simulink model "Closed_loop_response_PD_Controller"  (R2023a)
settings: Solver=FixedStepDiscrete  StartTime=0.0  StopTime=12  FixedStep=0.01  RelTol=1e-3  EnableMultiTasking=on
model workspace (MAT data in the model file):
  in = 90
undefined symbols (not defined in the file): DiscIntNeverNeededParam
libraries: M5Core_Library x2, simulink x1
settings Model: ExtModeTrigDuration=2  Creator=auw_a  LastModifiedBy=auw_a
settings OptimizationCC: EnhancedBackFolding=on  PassReuseOutputArgsAs=Individual arguments  ZeroExternalMemoryAtStartup=off  ZeroInternalMemoryAtStartup=off  MaxStackSize=64  OptimizeBlockOrder=speed  DifferentSizesBufferReuse=on  OptimizationCustomize=off  EfficientTunableParamExpr=on
settings DebuggingCC: ParameterOverflowMsg=none  ParameterTunabilityLossMsg=error
settings HardwareCC: ProdBitPerPointer=32  ProdBitPerSizeT=32  ProdBitPerPtrDiffT=32  ProdLargestAtomicInteger=Long  ProdLargestAtomicFloat=Double  ProdWordSize=32  ProdHWDeviceType=ARM Compatible->ARM Cortex
settings SFSimCC: MATLABDynamicMemAlloc=off
settings RTWCC: Description=Embedded Coder  SystemTargetFile=ert.tlc  HardwareBoard=ESP32-WROOM(Arduino Compatible)  TLCOptions="-aInlineSetEventsForThisBaseRateFcn=TLC_FALSE -aSuppressMultiTaskScheduler=TLC_FALSE  -aRateBasedStepFcn=0"  TemplateMakefile=ert_default_tmf  Toolchain=ESP32  BuildConfiguration=Faster Runs
settings CodeAppCC: ForceParamTrailComments=on  IgnoreCustomStorageClasses=off  OperatorAnnotations=on  SimulinkDataObjDesc=on  SFDataObjDesc=on  InsertBlockDesc=on
settings ERTTargetCC: SupportContinuousTime=on  SupportVariableSizeSignals=on  ExtModeTransport=3  ExtModeStaticAlloc=on  ExtModeAutomaticAllocSize=off  ExtModeStaticAllocSize=65536  ExtModeMexFile=ext_xcp  ExtModeIntrfLevel=Level2 - Open

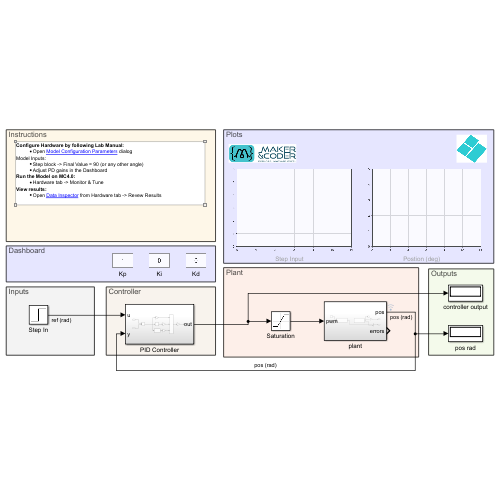
[thumbnail: Simulink's stored preview of the top-level diagram]
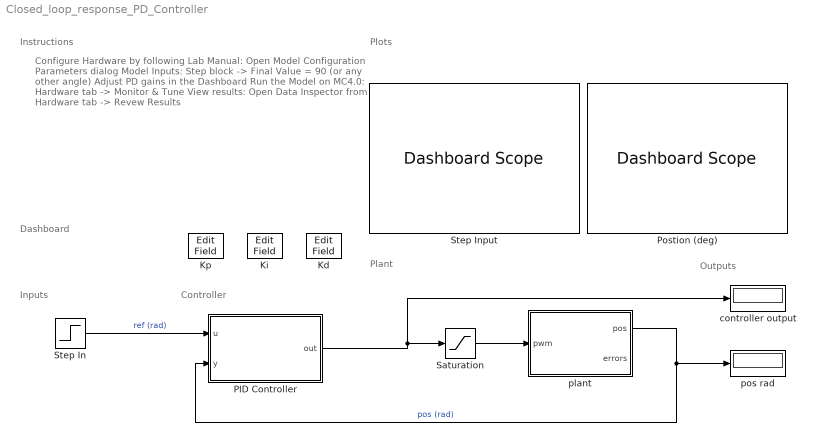
== system Closed_loop_response_PD_Controller ==
  note: Dashboard
  note: Outputs
  note: Inputs
  note: Controller
  note: Plant
  note: Plots
  note: Instructions
  note: Configure Hardware by following Lab Manual:
      | Open Model Configuration Parameters dialog
      | Model Inputs:
      | Step block -> Final Value = 90 (or any other angle)
      | Adjust PD gains in the Dashboard
      | Run the Model on MC4.0:
      | Hardware tab -> Monitor & Tune
      | View results:
      | Open Data Inspector from Hardware tab -> Revew Results
  Kd : EditField  LabelPosition=Hide  ShowInitialText=on  Alignment=Center
  Ki : EditField  LabelPosition=Hide  ShowInitialText=on  Alignment=Center
  Kp : EditField  LabelPosition=Hide  ShowInitialText=on  Alignment=Center
  PID Controller : Subsystem
  Postion (deg) : DashboardScope  Ymin=0  Ymax=5
  Saturation : Saturate  UpperLimit=127  LowerLimit=-127  OutDataTypeStr=int8
  Step In : Step  SampleTime=0.01
  Step Input : DashboardScope  Ymin=0  Ymax=6
  controller output : Display
  plant : Subsystem
  pos rad : Display
  wires:
  Saturation/1 -> plant/1(pwm)
  plant/1(pos) -> PID Controller/2(y), pos rad/1  "pos (rad)"
  Step In/1 -> PID Controller/1(u)  "ref (rad)"
  PID Controller/1(out) -> Saturation/1, controller output/1

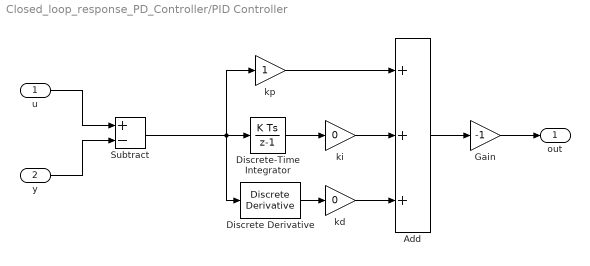
== system Closed_loop_response_PD_Controller/PID Controller ==
  u : Inport
  y : Inport  Port=2
  Add : Sum  Inputs=+++
  Discrete Derivative : simulink/Discrete/Discrete Derivative  gainval=1.0  ICPrevScaledInput=0.0  OutMin=[]  OutMax=[]  OutDataType=fixdt(1, 16)  OutScaling=2^-10  DoSatur=off
  Discrete-Time Integrator : DiscreteIntegrator  SampleTime=-1  ICPrevOutput=DiscIntNeverNeededParam  ICPrevScaledInput=DiscIntNeverNeededParam
  Gain : Gain  Gain=-1
  Subtract : Sum  Inputs=+-
  kd : Gain  Gain=0
  ki : Gain  Gain=0
  kp : Gain
  out : Outport
  wires:
  Discrete-Time Integrator/1 -> ki/1
  Subtract/1 -> Discrete Derivative/1, Discrete-Time Integrator/1, kp/1
  Discrete Derivative/1 -> kd/1
  ki/1 -> Add/2
  kp/1 -> Add/1
  kd/1 -> Add/3
  Add/1 -> Gain/1
  Gain/1 -> out/1
  y/1 -> Subtract/2
  u/1 -> Subtract/1

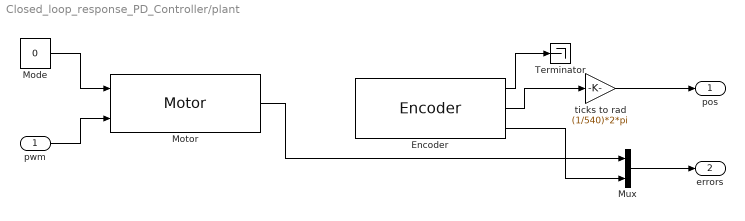
== system Closed_loop_response_PD_Controller/plant ==
  pwm : Inport
  Encoder : M5Core_Library/Encoder  M5_motor=2  s=0.01
  Mode : Constant  Value=0
  Motor : M5Core_Library/Motor  M5_motor=M2
  Mux : Mux  Inputs=2
  Terminator : Terminator
  ticks to rad : Gain  Gain=(1/540)*2*pi
  pos : Outport
  errors : Outport  Port=2
  wires:
  Motor/1 -> Mux/1
  Mux/1 -> errors/1
  Encoder/2 -> ticks to rad/1
  ticks to rad/1 -> pos/1
  Mode/1 -> Motor/1
  pwm/1 -> Motor/2
  Encoder/3 -> Mux/2
  Encoder/1 -> Terminator/1
